simulink model "AR4_robotv5"  (R2021a)
settings: Solver=VariableStepAuto  StartTime=0.0  StopTime=13.7896  RelTol=1e-3
undefined symbols (not defined in the file or in its folder): B, Levenberg, Marquardt, sigbuilder_block, Spline, X, Y, Z
libraries: sm_lib x612, nesl_utility x123, robotcorelib x28, simulink_extras x19, simulink x17, robotmaniplib x9
(part 14 of 14)

== matlab function AR4_robotv5/FIK13 ==
  data: H input; theta1 output; theta2 output; theta3 output; theta4 output; theta5 output; theta6 output; R60 output; O60 output; Oc0 output; X output; Y output; l1 output; l2 output; l3 output; l4 output; theta_B output; theta_C output; theta_D output; theta_E output; R63 output; RZ output; RY output; RX output
function [theta1, theta2, theta3, theta4, theta5, theta6, ...
          R60, O60, Oc0, X, Y, l1, l2, l3, l4, ...
          theta_B, theta_C, theta_D, theta_E, R63,RZ,RY,RX] = ...
          IK_AR4_withVerification(H)
% IK_AR4_withVerification Computes AR4 inverse kinematics with fixed orientation
% and selects the candidate that best reproduces the desired pose.
%
%   [theta1,theta2,theta3,theta4,theta5,theta6, R60, O60, Oc0, X, Y, l1, l2, l3, l4, ...
%    theta_B,theta_C,theta_D,theta_E,R63] = IK_AR4_withVerification(H)
%
%   Inputs:
%       H - 4x4 homogeneous transform (desired end-effector pose).
%           Both position and orientation are used for verification.
%
%   Outputs:
%       theta1 ... theta6 - Joint angles (degrees)
%       R60               - 3x3 rotation matrix extracted from H
%       O60               - 3x1 end-effector position from H
%       Oc0               - 3x1 wrist center position
%       X, Y              - Intermediate coordinates after base rotation
%       l1, l2, l3, l4    - Intermediate distances (mm)
%       theta_B ... theta_E - Auxiliary angles (deg)
%       R63               - 3x3 rotation from joint 3 to end-effector
%
%   AR4 Robot Geometry (mm):
%       a1 = 64.2; a2 = 305; a3 = 0;
%       d1 = 151.27; d4 = 225.04; d6 = 37.9;
%
%   The function computes two candidate solutions (elbow-up and elbow-down)
%   for joints 1–3 using the following conditions for θ₂:
%       if (xc > a1)
%           if (l4 > 0)
%               theta2 = theta_B + theta_C;
%           else
%               theta2 = theta_B + theta_C + 180;
%           end
%       else
%           theta2 = -(theta_B + theta_C);
%       end
%
%   Then, for each candidate, the wrist angles (θ₄, θ₅, θ₆) are computed using:
%
%       theta5 = atan2( sqrt(1 - r33^2), r33 );
%       if theta5 > 0, wc = 'F'; else, wc = 'N'; end
%       if theta5 > 0
%           theta4 = -rad2deg(atan2(-r23, r13));
%       else
%           theta4 = -rad2deg(atan2(r23, -r13));
%       end
%       if strcmp(wc, 'F') && rad2deg(atan2(sqrt(1 - r33^2), r33)) > 0
%           theta5 = rad2deg(atan2(sqrt(1 - r33^2), r33));
%       else
%           theta5 = rad2deg(atan2(sqrt(1 - r33^2), r33));
%       end
%       if theta5 > 0
%           theta6 = rad2deg(atan2(r32, -r31));
%       else
%           theta6 = rad2deg(atan2(-r32, r31));
%       end
%
%   Finally, the candidate with the smallest pose error (via forward kinematics)
%   is selected.
    
    %% 1) AR4 Geometry (mm)
    a1 = 64.2;
    a2 = 305;
    a3 = 0;        % Forearm length = 0 for AR4
    d1 = 151.27;
    d4 = 225.04;
    d6 = 84.832;

    %% 2) Extract Desired Pose from H
    R60 = H(1:3,1:3);  % Desired end-effector rotation
    O60 = H(1:3,4);    % Desired end-effector position

    % Compute wrist center: subtract d6 along the desired tool z-axis.
    % (Assuming the tool z-axis is given by R60(:,3))
    Oc0 = O60 - d6 * R60(:,3);
    xc = Oc0(1);
    yc = Oc0(2);
    zc = Oc0(3);

    %% 3) Inverse Position for Joints 1-3
    % Joint 1 (theta1)
    if abs(xc) < 1e-6
        theta1 = 0;
    else
        theta1 = atan2d(yc, xc);
    end

    % Rotate wrist center into joint 2's frame (remove effect of theta1)
    X =  xc*cosd(-theta1) - yc*sind(-theta1);
    Y =  yc*cosd(-theta1) + xc*sind(-theta1);

    % Distances:
    l1 = abs(X - a1);    % horizontal distance from base offset
    l4 = zc - d1;        % vertical offset from base height
    l2 = sqrt(l1^2 + l4^2);
    l3 = sqrt(d4^2 + a3^2);   % for AR4, l3 = d4

    % Auxiliary angles (in degrees)
    % Note: θ_B can be negative.
    theta_B = atan2d(l1, l4) ;
    theta_C = acosd((a2^2 + l2^2 - l3^2) / (2*a2*l2));
    theta_D = acosd((a2^2 + l3^2 - l2^2) / (2*a2*l3));
    theta_E = atan2d(a3, d4);   % typically 0 if a3 = 0

    % --- Candidate 1: Elbow-Up Branch ---
    if xc > a1
        if l4 > 0
            theta2A = theta_B - theta_C;
        else
            theta2A = theta_B - theta_C + 180;
        end
    else
        theta2A = -(theta_B + theta_C);
    end
    theta3A = 90 - (theta_D + theta_E);

    % --- Candidate 2: Elbow-Down Branch ---
    theta2B = theta_B - theta_C;
    theta3B = 90 + (theta_D + theta_E)-180;

    %% 4) For each candidate, compute wrist (Joints 4-6) using provided conditions.
    % We'll compute wrist angles from the forward kinematics of joints 1-3.
    % For candidate i, compute H30 from joints 1-3 then R63 = R30' * R60, then apply:
    % (The provided snippet for wrist angles)
    solutions = zeros(2,6);
    candidates = [theta2A, theta3A; theta2B, theta3B];
    for i = 1:2
        th1 = theta1;
        th2 = candidates(i,1);
        th3 = candidates(i,2);
        % Compute forward kinematics for joints 1-3:
        DH_3 = [ th1,         d1, a1, -90;
                 th2 - 90,    0,  a2,  0;
                 th3 + 180,   0,  a3,  90];
        A1 = computeDH(DH_3(1,:));
        A2 = computeDH(DH_3(2,:));
        A3 = computeDH(DH_3(3,:));
        temp = A1 * A2 * A3;
        R30 = temp(1:3,1:3);
        R63 = R30' * R60;  % Wrist orientation matrix

        % Extract elements of R63:
        r13 = R63(1,3);
        r23 = R63(2,3);
        r33 = R63(3,3);
        r31 = R63(3,1);
        r32 = R63(3,2);

        % Compute wrist angles:
        % theta5 preliminary (in radians, then deg)
        theta5_candidate = rad2deg(atan2(sqrt(1 - r33^2), r33));
        if theta5_candidate > 0
            wc = 'F'; % Flipped
        else
            wc = 'N'; % Normal
        end
        if theta5_candidate > 0
            theta4_candidate = -rad2deg(atan2(-r23, r13));
        else
            theta4_candidate = -rad2deg(atan2(r23, -r13));
        end
        % The following if-else for theta5 is redundant; we simply assign:
        theta5_candidate = rad2deg(atan2(sqrt(1 - r33^2), r33));
        if theta5_candidate > 0
            theta6_candidate = rad2deg(atan2(r32, -r31));
        else
            theta6_candidate = rad2deg(atan2(-r32, r31));
        end

        % Store candidate solution [theta1, theta2, theta3, theta4, theta5, theta6]
        solutions(i,:) = [th1, th2, th3, theta4_candidate, theta5_candidate, theta6_candidate];
    end

    %% 5) Verify candidates via forward kinematics and pick the best
    bestIdx = 1;
    bestError = inf;
    for i = 1:2
        cand = solutions(i,:);
        Hcand = forward_kinematics_AR4(cand(1), cand(2), cand(3), cand(4), cand(5), cand(6));
        err = measurePoseDifference(H, Hcand);
        if err < bestError
            bestError = err;
            bestIdx = i;
        end
    end

    bestSol = solutions(bestIdx,:);
    theta1 = bestSol(1);
    theta2 = bestSol(2);
    theta3 = bestSol(3);
    theta4 = bestSol(4);
    theta5 = bestSol(5);
    theta6 = bestSol(6);

    %% 6) Clean up near-zero values (optional)
    smallVal = 1e-6;
    if abs(theta1) < smallVal, theta1 = 0; end
    if abs(theta2) < smallVal, theta2 = 0; end
    if abs(theta3) < smallVal, theta3 = 0; end
    if abs(theta4) < smallVal, theta4 = 0; end
    if abs(theta5) < smallVal, theta5 = 0; end
    if abs(theta6) < smallVal, theta6 = 0; end

    %% 7) For completeness, compute R63 for output (from final solution)
    DH_3 = [theta1,        d1, a1, -90;
            theta2 - 90,   0,  a2,  0;
            theta3 + 180,  0,  a3,  90];
    A1 = computeDH(DH_3(1,:));
    A2 = computeDH(DH_3(2,:));
    A3 = computeDH(DH_3(3,:));
    temp = A1 * A2 * A3;
    R30 = temp(1:3,1:3);
    R63 = R30' * R60;
     %% 8) Extract RX, RY, RZ from R60 (Euler angles, ZYX convention)
    % R60 is the rotation matrix from the base to the end-effector
    % We'll extract Euler angles in ZYX order (RZ * RY * RX)
    R = R60;
    
    % Extract RY (pitch) angle
    RY_rad = atan2(-R(3,1), sqrt(R(1,1)^2 + R(2,1)^2));
    RY = rad2deg(RY_rad);
    
    % Check for gimbal lock (cos(RY) ≈ 0)
    if abs(cos(RY_rad)) > 1e-6
        % No gimbal lock
        RX_rad = atan2(R(3,2), R(3,3));
        RZ_rad = atan2(R(2,1), R(1,1));
    else
        % Gimbal lock case (RY ≈ ±90°)
        RX_rad = 0; % Arbitrary, can choose 0
        RZ_rad = atan2(R(1,2), R(2,2));
    end
    
    RX = rad2deg(RX_rad);
    RZ = rad2deg(RZ_rad);
end


%% ------------------------------------------------------------------------
function A = computeDH(dh)
    theta = dh(1);
    d     = dh(2);
    a     = dh(3);
    alpha = dh(4);
    A = [ cosd(theta), -sind(theta)*cosd(alpha),  sind(theta)*sind(alpha), a*cosd(theta);
          sind(theta),  cosd(theta)*cosd(alpha), -cosd(theta)*sind(alpha), a*sind(theta);
          0,            sind(alpha),              cosd(alpha),            d;
          0,            0,                        0,                      1];
end

%% ------------------------------------------------------------------------
function distVal = measurePoseDifference(Hdesired, Hactual)
    posDesired = Hdesired(1:3,4);
    posActual  = Hactual(1:3,4);
    dPos = norm(posDesired - posActual);
    Rdes = Hdesired(1:3,1:3);
    Ract = Hactual(1:3,1:3);
    Rerr = Rdes' * Ract;
    traceVal = (trace(Rerr) - 1) / 2;
    traceVal = max(-1, min(1, traceVal));
    orientErrorDeg = abs(rad2deg(acos(traceVal)));
    distVal = dPos + orientErrorDeg;
end

%% ------------------------------------------------------------------------
function Hfk = forward_kinematics_AR4(t1, t2, t3, t4, t5, t6)
    a1 = 64.2;
    a2 = 305;
    a3 = 0;
    d1 = 151.27;
    d4 = 225.04;
    d6 = 37.9;
    DH1 = [t1,       d1, a1, -90];
    DH2 = [t2-90,    0,  a2,   0];
    DH3 = [t3+180,   0,  a3,  90];
    DH4 = [t4,      d4,  0,  -90];
    DH5 = [t5,       0,  0,   90];
    DH6 = [t6,      d6,  0,    0];
    A1 = computeDH(DH1);
    A2 = computeDH(DH2);
    A3 = computeDH(DH3);
    A4 = computeDH(DH4);
    A5 = computeDH(DH5);
    A6 = computeDH(DH6);
    Hfk = A1 * A2 * A3 * A4 * A5 * A6;
end

== matlab function AR4_robotv5/circle3 ==
  data: u input; xd output; yd output; zd output; H output
function [xd, yd, zd, H] = Curved_Trajectory(u)
  
% Parameters
    radius = 200;          % Radius of the arc (mm)
    arc_angle = pi;       % Total arc angle (radians), pi = half-circle
    z_height = 400;       % Fixed height in Z (mm)
    T = 10;               % Time to complete the curve (seconds)

    % Clamp u within [0, T]
    u = min(max(u, 0), T);
    
    % Angle at time u
    theta = arc_angle * (u / T);  % From 0 to arc_angle

    % Center of arc (adjust as needed for your workspace)
    center_x = 100;
    center_y = 100;

    % Generate position along the arc
    xd = center_x + radius * cos(pi/2 - theta);  % Starts at bottom of arc
    yd = center_y + radius * sin(pi/2 - theta);
    zd = z_height;

    % No rotation
    R = eye(3);

    % Homogeneous transformation matrix
    H = [R, [xd; yd; zd]; 0 0 0 1];
end

== matlab function AR4_robotv5/MATLAB Function1 ==
  data: u input
function PlotTrajectoryFromFunction(u)
    % Simulates getting x, y, z from another function step-by-step
    % and shows the trajectory on a single figure

    % Example: arc trajectory
    total_points = 100;
    x_all = zeros(1, total_points);
    y_all = zeros(1, total_points);
    z_all = zeros(1, total_points);

    figure;
    hold on;
    grid on;
    axis equal;
    xlabel('X (mm)');
    ylabel('Y (mm)');
    zlabel('Z (mm)');
    title('Trajectory Accumulated in 3D');
    view(3);

    % Plot handle for updating
    trajPlot = plot3(NaN, NaN, NaN, 'b-', 'LineWidth', 2);

    for i = 1:total_points
        % Simulate getting point from another function
        t = linspace(0, pi, total_points);
      
% Parameters
    radius = 200;          % Radius of the arc (mm)
    arc_angle = pi;       % Total arc angle (radians), pi = half-circle
    z_height = 400;       % Fixed height in Z (mm)
    T = 10;               % Time to complete the curve (seconds)

    % Clamp u within [0, T]
    u = min(max(u, 0), T);
    
    % Angle at time u
    theta = arc_angle * (u / T);  % From 0 to arc_angle

    % Center of arc (adjust as needed for your workspace)
    center_x = 100;
    center_y = 100;

    % Generate position along the arc
    x = center_x + radius * cos(pi/2 - theta);  % Starts at bottom of arc
    y = center_y + radius * sin(pi/2 - theta);
    z= z_height;
        % Save to buffer
        x_all(i) = x;
        y_all(i) = y;
        z_all(i) = z;

        % Update plot
        set(trajPlot, 'XData', x_all(1:i), 'YData', y_all(1:i), 'ZData', z_all(1:i));
        drawnow;
        pause(0.01);  % optional: slow down to see drawing
    end

    % Optionally mark start and end
    plot3(x_all(1), y_all(1), z_all(1), 'go', 'MarkerSize', 10, 'LineWidth', 2);   % Start
    plot3(x_all(end), y_all(end), z_all(end), 'ro', 'MarkerSize', 10, 'LineWidth', 2); % End
end

== matlab function AR4_robotv5/MATLAB Function5 ==
  data: theta1 input; H output; theta2 input; theta3 input; theta4 input; theta5 input; theta6 input; X output; Y output; Z output; Rz output; Ry output; Rx output
function [H, X, Y, Z, Rz, Ry, Rx] = forward_kinematics_AR4(theta1, theta2, theta3, theta4, theta5, theta6)
% forward_kinematics_AR4 Computes the forward kinematics for the AR4 robot.
%
%   [H, X, Y, Z, Rz, Ry, Rx] = forward_kinematics_AR4(theta1, theta2, theta3, theta4, theta5, theta6)
%
%   Inputs:
%       theta1, theta2, theta3, theta4, theta5, theta6 - Joint angles (degrees)
%
%   Outputs:
%       H  - 4x4 homogeneous transformation matrix of the end-effector (mm)
%       X, Y, Z - End-effector position coordinates (mm)
%       Rz, Ry, Rx - End-effector orientation angles in degrees (ZYX Euler angles)
%
%   The AR4 robot parameters (in mm) used here are:
%       a1 = 64.2;   a2 = 305;    a3 = 0;
%       d1 = 151.27; d4 = 225.04; d6 = 37.9;
%
%   The DH parameters are defined as:
%       Joint 1: [theta1,         d1, a1, -90]
%       Joint 2: [theta2 - 90,     0,  a2,   0]
%       Joint 3: [theta3 + 180,    0,  a3,  90]
%       Joint 4: [theta4,         d4,  0,   -90]
%       Joint 5: [theta5,          0,  0,    90]
%       Joint 6: [theta6,         d6,  0,     0]

    %% Robot parameters
    a1 = 64.2;     a2 = 305;    a3 = 0;
    d1 = 151.27;   d4 = 225.04; d6 = 84.832;

    %% DH parameters
    DH1 = [theta1,       d1, a1, -90];
    DH2 = [theta2 - 90,  0,  a2,   0];
    DH3 = [theta3 + 180, 0,  a3,  90];
    DH4 = [theta4,       d4,  0,   -90];
    DH5 = [theta5,        0,  0,    90];
    DH6 = [theta6,       d6,  0,     0];

    %% Compute transformations
    A1 = computeDH(DH1);
    A2 = computeDH(DH2);
    A3 = computeDH(DH3);
    A4 = computeDH(DH4);
    A5 = computeDH(DH5);
    A6 = computeDH(DH6);

    H = A1 * A2 * A3 * A4 * A5 * A6;

    %% Extract position
    X = H(1,4);
    Y = H(2,4);
    Z = H(3,4);

    %% Extract orientation (ZYX Euler angles in degrees)
    R = H(1:3, 1:3);
    
    % Calculate Ry (pitch)
    Ry = atan2d(-R(3,1), sqrt(R(3,2)^2 + R(3,3)^2));
    
    % Check for gimbal lock (pitch near ±90°)
    if abs(abs(Ry) - 90) < eps
        % Gimbal lock case - set yaw to 0 and compute roll from alternate terms
        Rz = 0;
        Rx = atan2d(R(1,2), R(2,2));
    else
        % Normal case
        Rz = atan2d(R(2,1), R(1,1));
        Rx = atan2d(R(3,2), R(3,3));
    end
end

function A = computeDH(dh)
    theta = dh(1);
    d     = dh(2);
    a     = dh(3);
    alpha = dh(4);
    
    A = [cosd(theta), -sind(theta)*cosd(alpha),  sind(theta)*sind(alpha), a*cosd(theta);
         sind(theta),  cosd(theta)*cosd(alpha), -cosd(theta)*sind(alpha), a*sind(theta);
         0,            sind(alpha),             cosd(alpha),             d;
         0,            0,                       0,                       1];
end

== matlab function AR4_robotv5/Subsystem9/MATLAB Function4 ==
  data: theta1 input; H output; theta2 input; theta3 input; theta4 input; theta5 input; theta6 input; X output; Y output; Z output; Rz output; Ry output; Rx output
function [H, X, Y, Z, Rz, Ry, Rx] = forward_kinematics_AR4(theta1, theta2, theta3, theta4, theta5, theta6)
% forward_kinematics_AR4 Computes the forward kinematics for the AR4 robot.
%
%   [H, X, Y, Z, Rz, Ry, Rx] = forward_kinematics_AR4(theta1, theta2, theta3, theta4, theta5, theta6)
%
%   Inputs:
%       theta1, theta2, theta3, theta4, theta5, theta6 - Joint angles (degrees)
%
%   Outputs:
%       H  - 4x4 homogeneous transformation matrix of the end-effector (mm)
%       X, Y, Z - End-effector position coordinates (mm)
%       Rz, Ry, Rx - End-effector orientation angles in degrees (ZYX Euler angles)
%
%   The AR4 robot parameters (in mm) used here are:
%       a1 = 64.2;   a2 = 305;    a3 = 0;
%       d1 = 151.27; d4 = 225.04; d6 = 37.9;
%
%   The DH parameters are defined as:
%       Joint 1: [theta1,         d1, a1, -90]
%       Joint 2: [theta2 - 90,     0,  a2,   0]
%       Joint 3: [theta3 + 180,    0,  a3,  90]
%       Joint 4: [theta4,         d4,  0,   -90]
%       Joint 5: [theta5,          0,  0,    90]
%       Joint 6: [theta6,         d6,  0,     0]

    %% Robot parameters
    a1 = 64.2;     a2 = 305;    a3 = 0;
    d1 = 151.27;   d4 = 225.04; d6 = 84.832;

    %% DH parameters
    DH1 = [theta1,       d1, a1, -90];
    DH2 = [theta2 - 90,  0,  a2,   0];
    DH3 = [theta3 + 180, 0,  a3,  90];
    DH4 = [theta4,       d4,  0,   -90];
    DH5 = [theta5,        0,  0,    90];
    DH6 = [theta6,       d6,  0,     0];

    %% Compute transformations
    A1 = computeDH(DH1);
    A2 = computeDH(DH2);
    A3 = computeDH(DH3);
    A4 = computeDH(DH4);
    A5 = computeDH(DH5);
    A6 = computeDH(DH6);

    H = A1 * A2 * A3 * A4 * A5 * A6;

    %% Extract position
    X = H(1,4);
    Y = H(2,4);
    Z = H(3,4);

    %% Extract orientation (ZYX Euler angles in degrees)
    R = H(1:3, 1:3);
    
    % Calculate Ry (pitch)
    Ry = atan2d(-R(3,1), sqrt(R(3,2)^2 + R(3,3)^2));
    
    % Check for gimbal lock (pitch near ±90°)
    if abs(abs(Ry) - 90) < eps
        % Gimbal lock case - set yaw to 0 and compute roll from alternate terms
        Rz = 0;
        Rx = atan2d(R(1,2), R(2,2));
    else
        % Normal case
        Rz = atan2d(R(2,1), R(1,1));
        Rx = atan2d(R(3,2), R(3,3));
    end
end

function A = computeDH(dh)
    theta = dh(1);
    d     = dh(2);
    a     = dh(3);
    alpha = dh(4);
    
    A = [cosd(theta), -sind(theta)*cosd(alpha),  sind(theta)*sind(alpha), a*cosd(theta);
         sind(theta),  cosd(theta)*cosd(alpha), -cosd(theta)*sind(alpha), a*sind(theta);
         0,            sind(alpha),             cosd(alpha),             d;
         0,            0,                       0,                       1];
end

== matlab function AR4_robotv5/MATLAB Function2 ==
  data: theta1 input; H output; theta2 input; theta3 input; theta4 input; theta5 input; theta6 input; q output; Rz output; Ry output; Rx output
function [H, q, Rz, Ry, Rx] = forward_kinematics_AR4(theta1, theta2, theta3, theta4, theta5, theta6)
% forward_kinematics_AR4 Computes the forward kinematics for the AR4 robot.
%
%   [H, X, Y, Z, Rz, Ry, Rx] = forward_kinematics_AR4(theta1, theta2, theta3, theta4, theta5, theta6)
%
%   Inputs:
%       theta1, theta2, theta3, theta4, theta5, theta6 - Joint angles (degrees)
%
%   Outputs:
%       H  - 4x4 homogeneous transformation matrix of the end-effector (mm)
%       X, Y, Z - End-effector position coordinates (mm)
%       Rz, Ry, Rx - End-effector orientation angles in degrees (ZYX Euler angles)
%
%   The AR4 robot parameters (in mm) used here are:
%       a1 = 64.2;   a2 = 305;    a3 = 0;
%       d1 = 151.27; d4 = 225.04; d6 = 37.9;
%
%   The DH parameters are defined as:
%       Joint 1: [theta1,         d1, a1, -90]
%       Joint 2: [theta2 - 90,     0,  a2,   0]
%       Joint 3: [theta3 + 180,    0,  a3,  90]
%       Joint 4: [theta4,         d4,  0,   -90]
%       Joint 5: [theta5,          0,  0,    90]
%       Joint 6: [theta6,         d6,  0,     0]

    %% Robot parameters
    a1 = 64.2;     a2 = 305;    a3 = 0;
    d1 = 151.27;   d4 = 225.04; d6 = 84.832;

    %% DH parameters
    DH1 = [theta1,       d1, a1, -90];
    DH2 = [theta2 - 90,  0,  a2,   0];
    DH3 = [theta3 + 180, 0,  a3,  90];
    DH4 = [theta4,       d4,  0,   -90];
    DH5 = [theta5,        0,  0,    90];
    DH6 = [theta6,       d6,  0,     0];

    %% Compute transformations
    A1 = computeDH(DH1);
    A2 = computeDH(DH2);
    A3 = computeDH(DH3);
    A4 = computeDH(DH4);
    A5 = computeDH(DH5);
    A6 = computeDH(DH6);

    H = A1 * A2 * A3 * A4 * A5 * A6;

    %% Extract position
   
        q = [H(1,4); H(2,4); H(3,4)];  % ← Cartesian position vector

    

    %% Extract orientation (ZYX Euler angles in degrees)
    R = H(1:3, 1:3);
    
    % Calculate Ry (pitch)
    Ry = atan2d(-R(3,1), sqrt(R(3,2)^2 + R(3,3)^2));
    
    % Check for gimbal lock (pitch near ±90°)
    if abs(abs(Ry) - 90) < eps
        % Gimbal lock case - set yaw to 0 and compute roll from alternate terms
        Rz = 0;
        Rx = atan2d(R(1,2), R(2,2));
    else
        % Normal case c
        Rz = atan2d(R(2,1), R(1,1));
        Rx = atan2d(R(3,2), R(3,3));
    end
end

function A = computeDH(dh)
    theta = dh(1);
    d     = dh(2);
    a     = dh(3);
    alpha = dh(4);
    
    A = [cosd(theta), -sind(theta)*cosd(alpha),  sind(theta)*sind(alpha), a*cosd(theta);
         sind(theta),  cosd(theta)*cosd(alpha), -cosd(theta)*sind(alpha), a*sind(theta);
         0,            sind(alpha),             cosd(alpha),             d;
         0,            0,                       0,                       1];
end

== matlab function AR4_robotv5/MATLAB Function11 ==
  data: theta1 input; H output; theta2 input; theta3 input; theta4 input; theta5 input; theta6 input; q output; Rz output; Ry output; Rx output
function [H, q, Rz, Ry, Rx] = forward_kinematics_AR4(theta1, theta2, theta3, theta4, theta5, theta6)
% forward_kinematics_AR4 Computes the forward kinematics for the AR4 robot.
%
%   [H, X, Y, Z, Rz, Ry, Rx] = forward_kinematics_AR4(theta1, theta2, theta3, theta4, theta5, theta6)
%
%   Inputs:
%       theta1, theta2, theta3, theta4, theta5, theta6 - Joint angles (degrees)
%
%   Outputs:
%       H  - 4x4 homogeneous transformation matrix of the end-effector (mm)
%       X, Y, Z - End-effector position coordinates (mm)
%       Rz, Ry, Rx - End-effector orientation angles in degrees (ZYX Euler angles)
%
%   The AR4 robot parameters (in mm) used here are:
%       a1 = 64.2;   a2 = 305;    a3 = 0;
%       d1 = 151.27; d4 = 225.04; d6 = 37.9;
%
%   The DH parameters are defined as:
%       Joint 1: [theta1,         d1, a1, -90]
%       Joint 2: [theta2 - 90,     0,  a2,   0]
%       Joint 3: [theta3 + 180,    0,  a3,  90]
%       Joint 4: [theta4,         d4,  0,   -90]
%       Joint 5: [theta5,          0,  0,    90]
%       Joint 6: [theta6,         d6,  0,     0]

    %% Robot parameters
    a1 = 64.2;     a2 = 305;    a3 = 0;
    d1 = 151.27;   d4 = 225.04; d6 = 84.832;

    %% DH parameters
    DH1 = [theta1,       d1, a1, -90];
    DH2 = [theta2 - 90,  0,  a2,   0];
    DH3 = [theta3 + 180, 0,  a3,  90];
    DH4 = [theta4,       d4,  0,   -90];
    DH5 = [theta5,        0,  0,    90];
    DH6 = [theta6,       d6,  0,     0];

    %% Compute transformations
    A1 = computeDH(DH1);
    A2 = computeDH(DH2);
    A3 = computeDH(DH3);
    A4 = computeDH(DH4);
    A5 = computeDH(DH5);
    A6 = computeDH(DH6);

    H = A1 * A2 * A3 * A4 * A5 * A6;

    %% Extract position
   
        q = [H(1,4); H(2,4); H(3,4)];  % ← Cartesian position vector

    

    %% Extract orientation (ZYX Euler angles in degrees)
    R = H(1:3, 1:3);
    
    % Calculate Ry (pitch)
    Ry = atan2d(-R(3,1), sqrt(R(3,2)^2 + R(3,3)^2));
    
    % Check for gimbal lock (pitch near ±90°)
    if abs(abs(Ry) - 90) < eps
        % Gimbal lock case - set yaw to 0 and compute roll from alternate terms
        Rz = 0;
        Rx = atan2d(R(1,2), R(2,2));
    else
        % Normal case c
        Rz = atan2d(R(2,1), R(1,1));
        Rx = atan2d(R(3,2), R(3,3));
    end
end

function A = computeDH(dh)
    theta = dh(1);
    d     = dh(2);
    a     = dh(3);
    alpha = dh(4);
    
    A = [cosd(theta), -sind(theta)*cosd(alpha),  sind(theta)*sind(alpha), a*cosd(theta);
         sind(theta),  cosd(theta)*cosd(alpha), -cosd(theta)*sind(alpha), a*sind(theta);
         0,            sind(alpha),             cosd(alpha),             d;
         0,            0,                       0,                       1];
end
